simulink model "saturated_pitch_system"  (R2019b)
settings: Solver=VariableStepAuto  StartTime=0.0  StopTime=4  RelTol=1e-3
undefined symbols (not defined in the file or in its folder): G_theta_samples
libraries: cstblocks x5
settings Model: Creator=amirhossein  LastModifiedBy=amirhossein

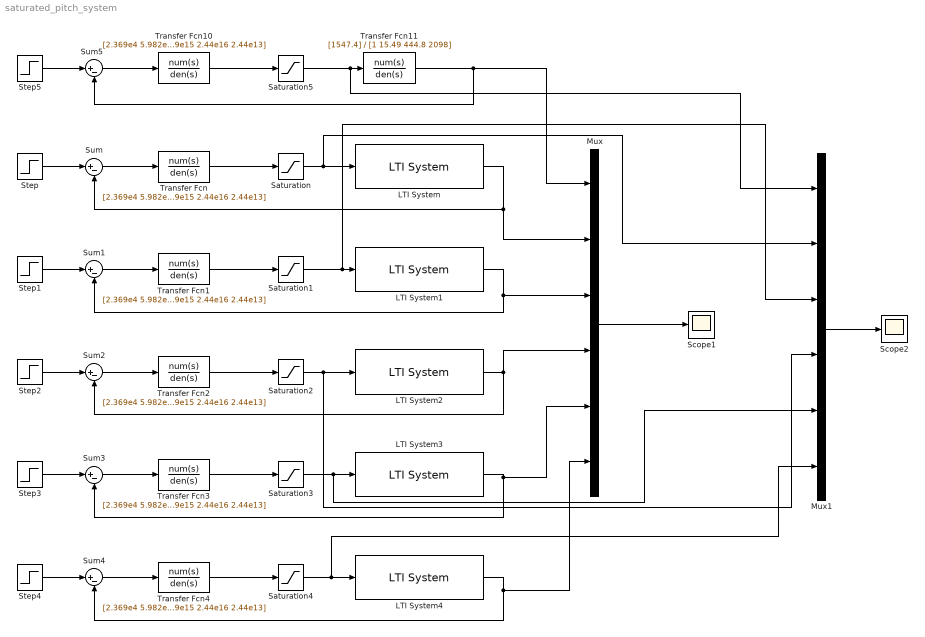
== system saturated_pitch_system ==
  LTI System : cstblocks/LTI System  sys=G_theta_samples(: , : , 1)  IC=[]
  LTI System1 : cstblocks/LTI System  sys=G_theta_samples(: , : , 2)  IC=[]
  LTI System2 : cstblocks/LTI System  sys=G_theta_samples(: , : , 3)  IC=[]
  LTI System3 : cstblocks/LTI System  sys=G_theta_samples(: , : , 4)  IC=[]
  LTI System4 : cstblocks/LTI System  sys=G_theta_samples(: , : , 5)  IC=[]
  Mux : Mux  Inputs=6
  Mux1 : Mux  Inputs=6
  Saturation{,1..5} (6 alike) : Saturate  UpperLimit=20  LowerLimit=-20
  Scope1 : Scope
  Scope2 : Scope
  Step{,1..5} (6 alike) : Step  SampleTime=0
  Sum{,1..5} (6 alike) : Sum  Inputs=|+-
  Transfer Fcn{,1..4,10} (6 alike) : TransferFcn  Numerator=[2.369e4 5.982e8 2.858e11 1.872e13 4.554e14 8.612e15 7.941e16 2.344e17]  Denominator=[1 2.715e4 6.056e7 3.819e10 3.997e12 2.165e14 4.539e15 2.44e16 2.44e13]
  Transfer Fcn11 : TransferFcn  Numerator=[1547.4]  Denominator=[1 15.49 444.8 2098]
  wires:
  Transfer Fcn/1 -> Saturation/1
  Saturation/1 -> Mux1/2, LTI System/1
  Sum/1 -> Transfer Fcn/1
  Step/1 -> Sum/1
  LTI System/1 -> Mux/2, Sum/2
  Transfer Fcn11/1 -> Sum5/2, Mux/1
  Transfer Fcn10/1 -> Saturation5/1
  Step5/1 -> Sum5/1
  Saturation5/1 -> Mux1/1, Transfer Fcn11/1
  Sum5/1 -> Transfer Fcn10/1
  Mux/1 -> Scope1/1
  Transfer Fcn1/1 -> Saturation1/1
  Saturation1/1 -> Mux1/3, LTI System1/1
  Step1/1 -> Sum1/1
  Sum1/1 -> Transfer Fcn1/1
  LTI System1/1 -> Mux/3, Sum1/2
  LTI System2/1 -> Mux/4, Sum2/2
  Step2/1 -> Sum2/1
  Transfer Fcn2/1 -> Saturation2/1
  Saturation2/1 -> Mux1/4, LTI System2/1
  Sum2/1 -> Transfer Fcn2/1
  LTI System3/1 -> Mux/5, Sum3/2
  Step3/1 -> Sum3/1
  Transfer Fcn3/1 -> Saturation3/1
  Saturation3/1 -> Mux1/5, LTI System3/1
  Sum3/1 -> Transfer Fcn3/1
  LTI System4/1 -> Mux/6, Sum4/2
  Step4/1 -> Sum4/1
  Transfer Fcn4/1 -> Saturation4/1
  Saturation4/1 -> Mux1/6, LTI System4/1
  Sum4/1 -> Transfer Fcn4/1
  Mux1/1 -> Scope2/1
